simulink model "as_quick_start"  (Simulink 7.8)
settings: Solver=ode1  StartTime=0.0  StopTime=inf  FixedStep=0.001  RelTol=1e-3
PostLoadFcn:
  | qc_set_target_type(getConfigSet(bdroot, 'QUARC Default Target Configuration'));
undefined symbols (not defined in the file): HIL, qc_get_step_size
libraries: quarc_library x8, simulink x3
settings Model: Creator=DCrymble  LastModifiedBy=pmartin  SimulationMode=external  ExtModeTrigDuration=50000
settings SolverCC: PositivePriorityOrder=on
settings OptimizationCC: InitFltsAndDblsToZero=on
settings DebuggingCC: SaveWithParameterizedLinksMsg=none  MultiTaskDSMMsg=warning  MultiTaskCondExecSysMsg=none  FcnCallInpInsideContextMsg=Use local settings  StrictBusMsg=None
settings RTWCC: SystemTargetFile=quarc_windows.tlc  TemplateMakefile=quarc_default_tmf  Description=QUARC Win32 Target  ProcessScript=quarc_windows_make_rtw_hook
settings STFCustomTargetCC: TargetPreCompLibLocation=C:\PROGRA~2\QUARC\lib\2012b\windows\release  SystemTargetFile=quarc_windows.tlc
settings GRTTargetCC: TargetPreCompLibLocation=C:\PROGRA~2\QUARC\lib\2012b\windows\release  ParMdlRefBuildCompliant=off  CompOptLevelCompliant=off  ConcurrentExecutionCompliant=off  MatFileLogging=off  ExtMode=on  ExtModeMexFile=quarc_comm

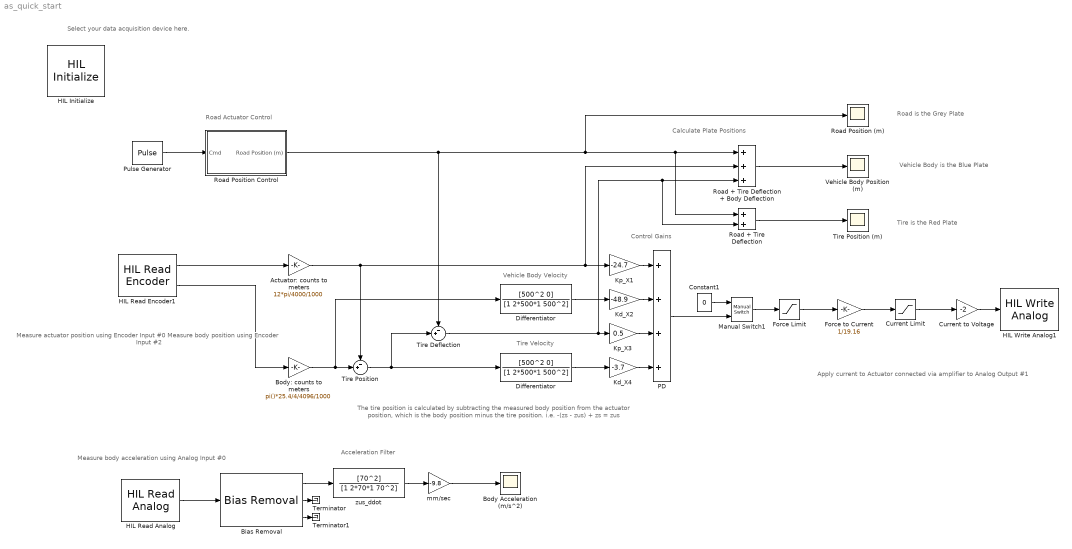
== system as_quick_start ==
  note: Measure actuator position using Encoder Input  #0
      | Measure body position using Encoder Input #2
  note: Select your data acquisition device here.
  note: Control Gains
  note: Vehicle Body Velocity
  note: Tire Velocity
  note: Road Actuator Control
  note: Calculate Plate Positions
  note: Measure body acceleration using Analog Input #0
  note: Acceleration Filter
  note: Apply current to Actuator connected via amplifier to Analog Output #1
  note: Road is the Grey Plate
  note: Vehicle Body is the Blue Plate
  note: Tire is the Red Plate
  note: The tire position is calculated by subtracting the measured body position from
      | the actuator position, which is the body position minus the tire position.
      | i.e. -(zs - zus) + zs = zus
  Actuator: counts to meters : Gain  Gain=12*pi/4000/1000
  Bias Removal : quarc_library/Discrete/Bias Removal  start_time=0  end_time=.099  switch_id=0  sample_time=qc_get_step_size
  Body Acceleration (m/s^2) : Scope
      settings: YMin=-2.5  YMax=2.25  MaxDataPoints=300000
  Body: counts to meters : Gain  Gain=pi()*25.4/4/4096/1000
  Constant1 : Constant  Value=0
  Current Limit : Saturate  UpperLimit=5  LowerLimit=-5
  Current to Voltage : Gain  Gain=-2
  Differentiator : TransferFcn  Numerator=[500^2 0]  Denominator=[1 2*500*1 500^2]
  "Differentiator " : TransferFcn  Numerator=[500^2 0]  Denominator=[1 2*500*1 500^2]
  Force Limit : Saturate  UpperLimit=39.2  LowerLimit=-39.2
  Force to Current : Gain  Gain=1/19.16
  HIL Initialize : quarc_library/Data Acquisition/Generic/Configuration/HIL Initialize  Priority=-99  object_name=HIL-1  board_type=q8_usb  board_number=0  board_options=update_rate=normal;decimation=1  exclusive=off  active=off  hardware_clocks=[0:2]  clock_modes=[]  initial_clock_frequencies=[]  set_clock_params_at_start=off  set_clock_params_at_switch_in=off  set_clock_frequencies_at_start=off  set_clock_frequencies_at_switch_in=off  analog_input_channels=[0:7]  analog_input_maximums=10  analog_input_minimums=-10  set_analog_input_params_at_start=on  set_analog_input_params_at_switch_in=off  analog_output_channels=[0:7]  analog_output_maximums=10  analog_output_minimums=-10  initial_analog_outputs=[0]  final_analog_outputs=[0]  watchdog_analog_outputs=0  set_analog_output_params_at_start=on  set_analog_output_params_at_switch_in=off  set_analog_outputs_at_start=on  set_analog_outputs_at_switch_in=off  set_analog_outputs_at_terminate=on  set_analog_outputs_at_switch_out=off  set_analog_outputs_on_watchdog=off  digital_input_channels=[]  digital_output_channels=[0:4]  digital_output_configuration=[]  initial_digital_outputs=[0 0 0 0 1]  final_digital_outputs=[1 1 1 1 0]  watchdog_digital_outputs=[0]  set_digital_output_params_at_start=off  set_digital_output_params_at_switch_in=off  set_digital_outputs_at_start=on  set_digital_outputs_at_switch_in=on  set_digital_outputs_at_terminate=on  set_digital_outputs_at_switch_out=off  set_digital_outputs_on_watchdog=off  encoder_channels=[0:7]  quadrature=[4]  encoder_filter_frequency=[]  initial_encoder_counts=[0]  set_encoder_params_at_start=on  set_encoder_params_at_switch_in=off  set_encoder_counts_at_start=on  set_encoder_counts_at_switch_in=off  pwm_channels=[0:7]  pwm_modes=0  pwm_frequency=99.532799999999995e6/4095  pwm_configuration=[0]  pwm_alignment=[0]  pwm_polarity=[1]  pwm_leading_deadband=[0]  pwm_trailing_deadband=[0]  initial_pwm_outputs=[0]  final_pwm_outputs=[0]  watchdog_pwm_outputs=[0]  set_pwm_params_at_start=on  set_pwm_params_at_switch_in=off  set_pwm_outputs_at_start=on  set_pwm_outputs_at_switch_in=off  set_pwm_outputs_at_terminate=on  set_pwm_outputs_at_switch_out=off  set_pwm_outputs_on_watchdog=off  other_output_channels=[]  initial_other_outputs=[]  final_other_outputs=[]  watchdog_other_outputs=[]  set_other_outputs_at_start=off  set_other_outputs_at_switch_in=off  set_other_outputs_at_terminate=off  set_other_outputs_at_switch_out=off  set_other_outputs_on_watchdog=off
  HIL Read Analog : quarc_library/Data Acquisition/Generic/Immediate I//O/HIL Read Analog  object_name=HIL-1  channels=0  sample_time=qc_get_step_size  active=on  vector_output=off
  HIL Read Encoder1 : quarc_library/Data Acquisition/Generic/Immediate I//O/HIL Read Encoder  object_name=HIL-1  channels=[0, 2]  sample_time=qc_get_step_size  active=on  vector_output=off  data_type_mode=Inherit via back propagation  data_type=double
  HIL Write Analog1 : quarc_library/Data Acquisition/Generic/Immediate I//O/HIL Write Analog  object_name=HIL-1  channels=0  sample_time=-1  active=off  vector_input=on
  Kd_X2 : Gain  Gain=-48.9
  Kd_X4 : Gain  Gain=-3.7
  Kp_X1 : Gain  Gain=-24.7
  Kp_X3 : Gain  Gain=0.5
  Manual Switch1 : simulink/Signal Routing/Manual Switch  sw=0  action=0  varsize=off
  PD : Sum  Inputs=++++
  Pulse Generator : DiscretePulseGenerator  PulseType=Time based  Amplitude=0.02  Period=3  PulseWidth=50  PhaseDelay=.1
  Road + Tire Deflection : Sum  Inputs=2  SaturateOnIntegerOverflow=on  InputSameDT=on  OutDataTypeStr=Inherit: Same as first input
  Road + Tire Deflection + Body Deflection : Sum  Inputs=3  SaturateOnIntegerOverflow=on  InputSameDT=on  OutDataTypeStr=Inherit: Same as first input
  Road Position (m) : Scope
      settings: YMin=-0.0225  YMax=0.0325  SaveName=ScopeData6  MaxDataPoints=300000
  Road Position Control : Subsystem
  Terminator : Terminator
  Terminator1 : Terminator
  Tire Deflection : Sum  Inputs=-+|
  Tire Position : Sum  Inputs=-+|
  Tire Position (m) : Scope
      settings: YMin=-0.0225  YMax=0.0325  SaveName=ScopeData3  MaxDataPoints=300000
  Vehicle Body Position (m) : Scope
      settings: YMin=-0.0225  YMax=0.0325  SaveName=ScopeData2  MaxDataPoints=300000
  mm/sec : Gain  Gain=-9.8
  zus_ddot : TransferFcn  Numerator=[70^2]  Denominator=[1 2*70*1 70^2]
  wires:
  Manual Switch1/1 -> Force Limit/1
  Constant1/1 -> Manual Switch1/1
  Road + Tire Deflection + Body Deflection/1 -> Vehicle Body Position (m)/1
  Road + Tire Deflection/1 -> Tire Position (m)/1
  Tire Deflection/1 -> Road + Tire Deflection + Body Deflection/3, Road + Tire Deflection/2, Kp_X3/1
  Actuator: counts to meters/1 -> Tire Position/1, Kp_X1/1, Road + Tire Deflection + Body Deflection/2
  HIL Read Encoder1/2 -> Body: counts to meters/1
  Current Limit/1 -> Current to Voltage/1
  Force to Current/1 -> Current Limit/1
  Current to Voltage/1 -> HIL Write Analog1/1
  Tire Position/1 -> Tire Deflection/2, "Differentiator "/1
  HIL Read Encoder1/1 -> Actuator: counts to meters/1
  Differentiator/1 -> Kd_X2/1
  "Differentiator "/1 -> Kd_X4/1
  Body: counts to meters/1 -> Differentiator/1, Tire Position/2
  Road Position Control/1(Road Position (m)) -> Tire Deflection/1, Road + Tire Deflection + Body Deflection/1, Road + Tire Deflection/1, Road Position (m)/1
  PD/1 -> Manual Switch1/2
  Force Limit/1 -> Force to Current/1
  Kp_X1/1 -> PD/1
  Kd_X2/1 -> PD/2
  Kp_X3/1 -> PD/3
  Kd_X4/1 -> PD/4
  HIL Read Analog/1 -> Bias Removal/1
  Bias Removal/1 -> zus_ddot/1
  zus_ddot/1 -> mm/sec/1
  mm/sec/1 -> Body Acceleration (m/s^2)/1
  Bias Removal/2 -> Terminator/1
  Bias Removal/3 -> Terminator1/1
  Pulse Generator/1 -> Road Position Control/1(Cmd)

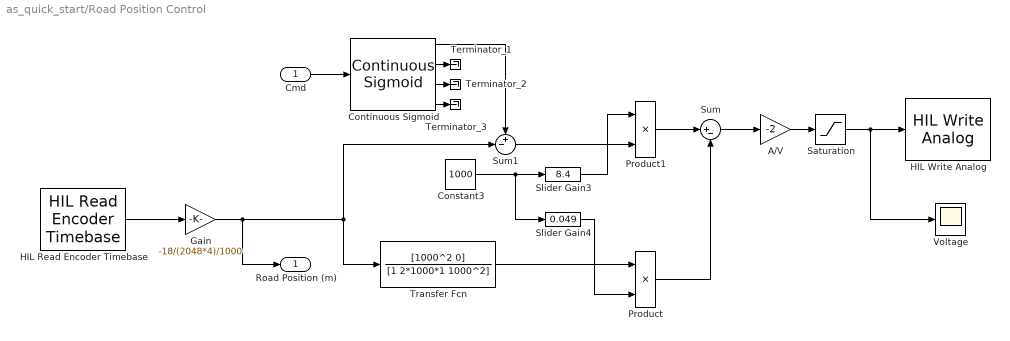
== system as_quick_start/Road Position Control ==
  Cmd : Inport
  A/V : Gain  Gain=-2
  Constant3 : Constant  Value=1000
  Continuous Sigmoid : quarc_library/Sources/Sigmoids/Continuous Sigmoid  params_source=Internal (dialog parameters)  max_velocity=.6/3  max_acceleration=20  initial_position=0  initial_velocity=0  hold_off=0.5  input_sample_time=-1  output_sample_time=qc_get_step_size
  Gain : Gain  Gain=-18/(2048*4)/1000
  HIL Read Encoder Timebase : quarc_library/Data Acquisition/Generic/Timebases/HIL Read Encoder Timebase  object_name=HIL-1  clock=[0]  channels=1  samples_in_buffer=max(ceil(1/qc_get_step_size), 1)  active=on  vector_output=on  data_type_mode=Inherit via back propagation  data_type=double
  HIL Write Analog : quarc_library/Data Acquisition/Generic/Immediate I//O/HIL Write Analog  object_name=HIL-1  channels=1  sample_time=-1  active=off  vector_input=on
  Product : Product  RndMeth=Zero
  Product1 : Product  RndMeth=Zero
  Saturation : Saturate  UpperLimit=10  LowerLimit=-10
  Slider Gain3 : simulink/Math Operations/Slider Gain  low=0  gain=8.4  high=70
  Slider Gain4 : simulink/Math Operations/Slider Gain  low=0  gain=0.049  high=0.1
  Sum : Sum  Inputs=|+-
  Sum1 : Sum  Inputs=+-|
  Terminator_1 : Terminator
  Terminator_2 : Terminator
  Terminator_3 : Terminator
  Transfer Fcn : TransferFcn  Numerator=[1000^2 0]  Denominator=[1 2*1000*1 1000^2]
  Voltage : Scope
      settings: TimeRange=1  YMin=-10.5  YMax=-9.5
  Road Position (m) : Outport
  wires:
  A/V/1 -> Saturation/1
  Constant3/1 -> Slider Gain4/1, Slider Gain3/1
  HIL Read Encoder Timebase/1 -> Gain/1
  Saturation/1 -> HIL Write Analog/1, Voltage/1
  Sum/1 -> A/V/1
  Gain/1 -> Road Position (m)/1, Transfer Fcn/1, Sum1/2
  Transfer Fcn/1 -> Product/1
  Slider Gain3/1 -> Product1/1
  Sum1/1 -> Product1/2
  Product1/1 -> Sum/1
  Slider Gain4/1 -> Product/2
  Product/1 -> Sum/2
  Continuous Sigmoid/2 -> Terminator_1/1
  Continuous Sigmoid/3 -> Terminator_2/1
  Continuous Sigmoid/4 -> Terminator_3/1
  Continuous Sigmoid/1 -> Sum1/1
  Cmd/1 -> Continuous Sigmoid/1
